simulink model "sim4"  (R2022b)
settings: Solver=VariableStepAuto  StartTime=0.0  StopTime=120  RelTol=1e-3
values from neighbouring files (symbols this model uses):
  A_int = [A zeros(4,1); zeros(1,5)]    [main.m]
  B_int = [B; 0 0]    [main.m]
  C_int = eye(5)    [main.m]
  D_int = zeros(5,2)    [main.m]
  Klqri = lqr(Ai, Bi, Qi, Ri)    [main.m]
libraries: simulink x5
settings Model: Creator=augusto  LastModifiedBy=augusto

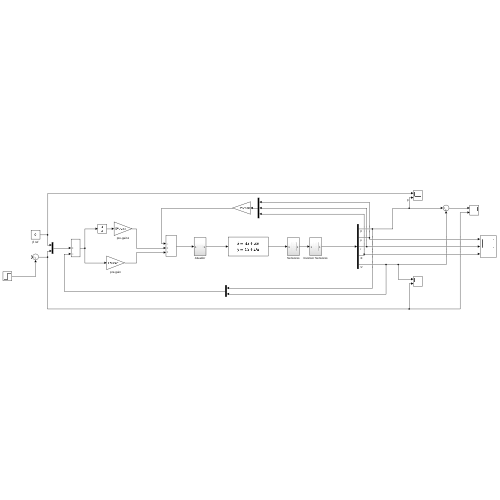
[thumbnail: Simulink's stored preview of the top-level diagram]
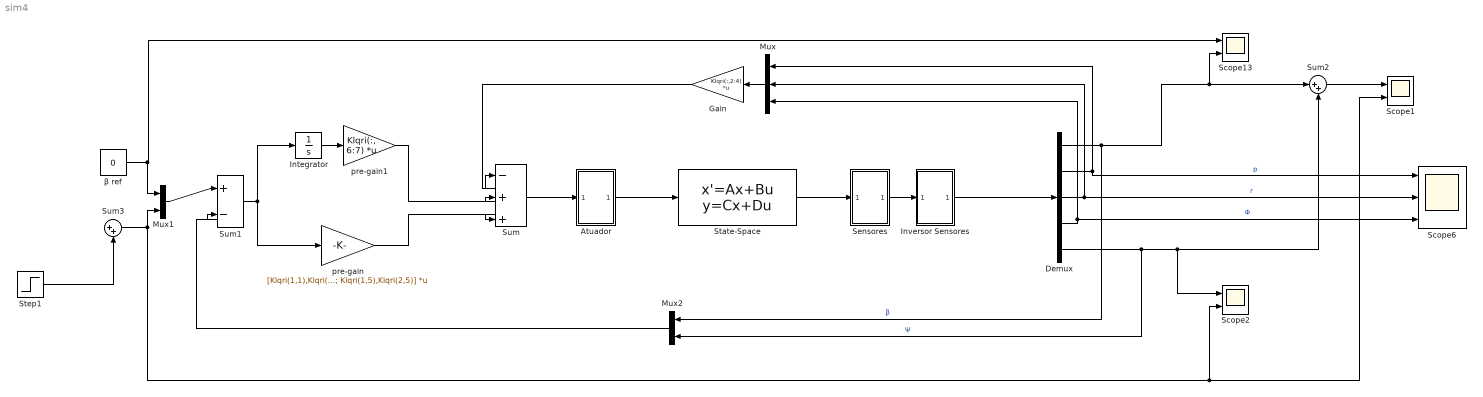
== system sim4 ==
  Atuador : Subsystem
  Demux : Demux  Outputs=5
  Gain : Gain  Gain=Klqri(:,2:4)  Multiplication=Matrix(K*u) (u vector)
  Integrator : Integrator
  Inversor Sensores : Subsystem
  Mux : Mux  Inputs=3
  Mux1 : Mux  Inputs=2
  Mux2 : Mux  Inputs=2
  Scope1 : Scope  NumInputPorts=2
  Scope13 : Scope  NumInputPorts=2
  Scope2 : Scope  NumInputPorts=2
  Scope6 : Scope  NumInputPorts=3
  Sensores : Subsystem
  State-Space : StateSpace  A=A_int  B=B_int  C=C_int  D=D_int  InitialCondition=0
  Step1 : Step  After=deg2rad(90)  SampleTime=0
  Sum : Sum  Inputs=|-++
  Sum1 : Sum  Inputs=|+-
  Sum2 : Sum  Inputs=|++
  Sum3 : Sum  Inputs=|++
  pre-gain : Gain  Gain=[Klqri(1,1),Klqri(2,1); Klqri(1,5),Klqri(2,5)]  Multiplication=Matrix(K*u) (u vector)
  pre-gain1 : Gain  Gain=Klqri(:, 6:7)  Multiplication=Matrix(K*u) (u vector)
  β ref : Constant  Value=0
  wires:
  Demux/1 -> Mux2/1, Scope13/2, Sum2/1  "β"
  Demux/5 -> Mux2/2, Sum2/2, Scope2/1  "Ψ"
  Sum2/1 -> Scope1/1
  Sum1/1 -> Integrator/1, pre-gain/1
  Demux/3 -> Mux/2, Scope6/2  "r"
  Demux/2 -> Mux/1, Scope6/1  "p"
  Demux/4 -> Mux/3, Scope6/3  "Φ"
  Mux1/1 -> Sum1/1
  Mux2/1 -> Sum1/2
  Integrator/1 -> pre-gain1/1
  Mux/1 -> Gain/1
  pre-gain/1 -> Sum/3
  pre-gain1/1 -> Sum/2
  Gain/1 -> Sum/1
  β ref/1 -> Mux1/1, Scope13/1
  Sum3/1 -> Scope1/2, Scope2/2, Mux1/2
  Step1/1 -> Sum3/2
  Sum/1 -> Atuador/1(In1)
  Atuador/1(Out1) -> State-Space/1
  Sensores/1(Out2) -> Inversor Sensores/1(In2)
  State-Space/1 -> Sensores/1(In2)
  Inversor Sensores/1(Out2) -> Demux/1

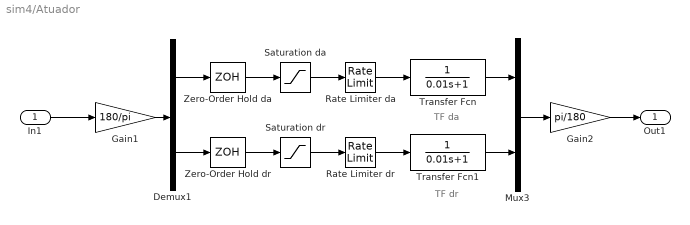
== system sim4/Atuador ==
  note: TF dr
  note: TF da
  In1 : Inport
  Demux1 : Demux  Outputs=2
  Gain1 : Gain  Gain=180/pi
  Gain2 : Gain  Gain=pi/180
  Mux3 : Mux  Inputs=2
  Rate Limiter dr : RateLimiter  RisingSlewLimit=60  FallingSlewLimit=-60  SampleTimeMode=inherited
  Rate Limiter da : RateLimiter  RisingSlewLimit=60  FallingSlewLimit=-60  SampleTimeMode=inherited
  Saturation da : Saturate  UpperLimit=30  LowerLimit=-30
  Saturation dr : Saturate  UpperLimit=30  LowerLimit=-30
  Transfer Fcn : TransferFcn  Denominator=[0.01 1]
  Transfer Fcn1 : TransferFcn  Denominator=[0.01 1]
  Zero-Order Hold da : ZeroOrderHold  SampleTime=1/40
  Zero-Order Hold dr : ZeroOrderHold  SampleTime=1/40
  Out1 : Outport
  wires:
  Saturation dr/1 -> Rate Limiter dr/1
  Gain2/1 -> Out1/1
  Demux1/2 -> Zero-Order Hold dr/1
  Demux1/1 -> Zero-Order Hold da/1
  Rate Limiter dr/1 -> Transfer Fcn1/1
  Transfer Fcn/1 -> Mux3/1
  Rate Limiter da/1 -> Transfer Fcn/1
  Zero-Order Hold da/1 -> Saturation da/1
  Saturation da/1 -> Rate Limiter da/1
  Transfer Fcn1/1 -> Mux3/2
  Gain1/1 -> Demux1/1
  Mux3/1 -> Gain2/1
  In1/1 -> Gain1/1
  Zero-Order Hold dr/1 -> Saturation dr/1

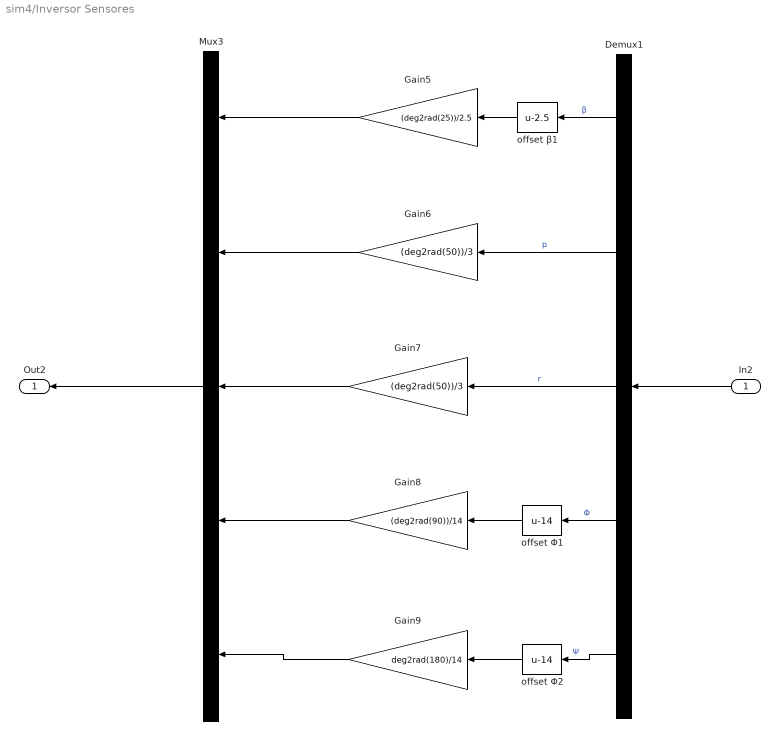
== system sim4/Inversor Sensores ==
  In2 : Inport
  Demux1 : Demux  Outputs=5
  Gain5 : Gain  Gain=(deg2rad(25))/2.5
  Gain6 : Gain  Gain=(deg2rad(50))/3
  Gain7 : Gain  Gain=(deg2rad(50))/3
  Gain8 : Gain  Gain=(deg2rad(90))/14
  Gain9 : Gain  Gain=deg2rad(180)/14
  Mux3 : Mux  Inputs=5
  offset Φ1 : Bias  Bias=-14  SaturateOnIntegerOverflow=off
  offset Φ2 : Bias  Bias=-14  SaturateOnIntegerOverflow=off
  offset β1 : Bias  Bias=-2.5  SaturateOnIntegerOverflow=off
  Out2 : Outport
  wires:
  Mux3/1 -> Out2/1
  In2/1 -> Demux1/1
  Demux1/1 -> offset β1/1  "β"
  Demux1/2 -> Gain6/1  "p"
  Demux1/3 -> Gain7/1  "r"
  Demux1/4 -> offset Φ1/1  "Φ"
  Demux1/5 -> offset Φ2/1  "Ψ"
  offset β1/1 -> Gain5/1
  Gain5/1 -> Mux3/1
  Gain6/1 -> Mux3/2
  offset Φ1/1 -> Gain8/1
  Gain8/1 -> Mux3/4
  offset Φ2/1 -> Gain9/1
  Gain9/1 -> Mux3/5
  Gain7/1 -> Mux3/3

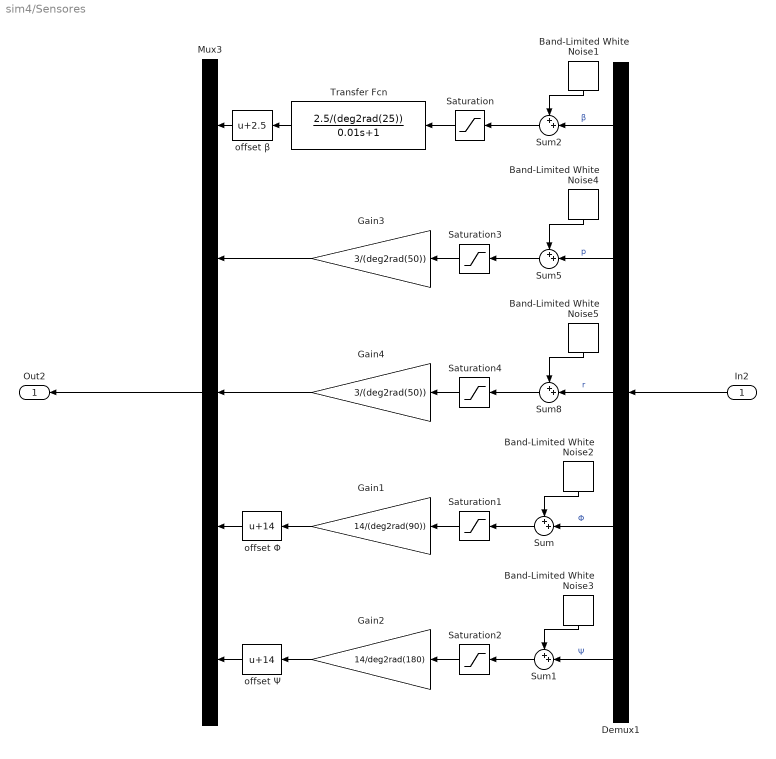
== system sim4/Sensores ==
  In2 : Inport
  Band-Limited White Noise1 : simulink/Sources/Band-Limited White Noise  Cov=noise_power_betha  Ts=10/1000  seed=[123]
  Band-Limited White Noise2 : simulink/Sources/Band-Limited White Noise  Cov=noise_power_rol  Ts=1/40  seed=[123]
  Band-Limited White Noise3 : simulink/Sources/Band-Limited White Noise  Cov=noise_power_yaw  Ts=1/40  seed=[123]
  Band-Limited White Noise4 : simulink/Sources/Band-Limited White Noise  Cov=noise_power_ang_vel  Ts=1/40  seed=[123]
  Band-Limited White Noise5 : simulink/Sources/Band-Limited White Noise  Cov=noise_power_ang_vel  Ts=1/40  seed=[123]
  Demux1 : Demux  Outputs=5
  Gain1 : Gain  Gain=14/(deg2rad(90))
  Gain2 : Gain  Gain=14/deg2rad(180)
  Gain3 : Gain  Gain=3/(deg2rad(50))
  Gain4 : Gain  Gain=3/(deg2rad(50))
  Mux3 : Mux  Inputs=5
  Saturation : Saturate  UpperLimit=deg2rad(25)  LowerLimit=-deg2rad(25)
  Saturation1 : Saturate  UpperLimit=deg2rad(90)  LowerLimit=-deg2rad(90)
  Saturation2 : Saturate  UpperLimit=deg2rad(360)  LowerLimit=0
  Saturation3 : Saturate  UpperLimit=deg2rad(50)  LowerLimit=-deg2rad(50)
  Saturation4 : Saturate  UpperLimit=deg2rad(50)  LowerLimit=-deg2rad(50)
  Sum{,1..2,5,8} (5 alike) : Sum  Inputs=++|
  Transfer Fcn : TransferFcn  Numerator=2.5/(deg2rad(25))  Denominator=[0.01 1]
  offset Φ : Bias  Bias=14  SaturateOnIntegerOverflow=off
  offset Ψ : Bias  Bias=14  SaturateOnIntegerOverflow=off
  offset β : Bias  Bias=2.5  SaturateOnIntegerOverflow=off
  Out2 : Outport
  wires:
  Saturation4/1 -> Gain4/1
  Saturation/1 -> Transfer Fcn/1
  Saturation2/1 -> Gain2/1
  Saturation1/1 -> Gain1/1
  Mux3/1 -> Out2/1
  In2/1 -> Demux1/1
  Demux1/1 -> Sum2/2  "β"
  Saturation3/1 -> Gain3/1
  offset β/1 -> Mux3/1
  Gain1/1 -> offset Φ/1
  offset Φ/1 -> Mux3/4
  Sum/1 -> Saturation1/1
  Demux1/4 -> Sum/2  "Φ"
  Band-Limited White Noise2/1 -> Sum/1
  offset Ψ/1 -> Mux3/5
  Gain2/1 -> offset Ψ/1
  Band-Limited White Noise3/1 -> Sum1/1
  Demux1/5 -> Sum1/2  "Ψ"
  Sum1/1 -> Saturation2/1
  Sum8/1 -> Saturation4/1
  Demux1/3 -> Sum8/2  "r"
  Band-Limited White Noise5/1 -> Sum8/1
  Gain4/1 -> Mux3/3
  Demux1/2 -> Sum5/2  "p"
  Sum5/1 -> Saturation3/1
  Gain3/1 -> Mux3/2
  Band-Limited White Noise4/1 -> Sum5/1
  Sum2/1 -> Saturation/1
  Band-Limited White Noise1/1 -> Sum2/1
  Transfer Fcn/1 -> offset β/1
